simulink model "Saucer_4dof"  (R2015b)
settings: Solver=ode4  StartTime=0.0  StopTime=tsim  FixedStep=0.01  RelTol=1e-3
values from neighbouring files (symbols this model uses):
  eta_init = zeros(4,1)    [run_Saucer_4dof.m]
  nu_init = zeros(4,1)    [run_Saucer_4dof.m]
libraries: simulink x1
settings Model: Creator=mclab  LastModifiedBy=Rotem
settings DataIOCC: SaveFormat=Array
settings DebuggingCC: SolverPrmCheckMsg=warning
settings HardwareCC: ProdBitPerPointer=32  ProdLargestAtomicFloat=None  ProdIntDivRoundTo=Undefined  ProdEndianess=Unspecified  ProdWordSize=32  ProdHWDeviceType=32-bit Generic
settings RTWCC: SystemTargetFile=NIVeriStand_VxWorks.tlc  TemplateMakefile=NIVeriStand_VxWorks.tmf  Description=NI VeriStand VxWorks Real-Time Target for Release 2007b or later
settings STFCustomTargetCC: ConcurrentExecutionCompliant=off  MatFileLogging=on  MATLABClassNameForMDSCustomization=Simulink.SoftwareTarget.TargetSpecificTriggerConfigurationBase  CPPClassGenCompliant=off  SystemTargetFile=NIVeriStand_VxWorks.tlc
settings ConfigComp: CovModelRefEnable=Off  CovSFcnEnable=off

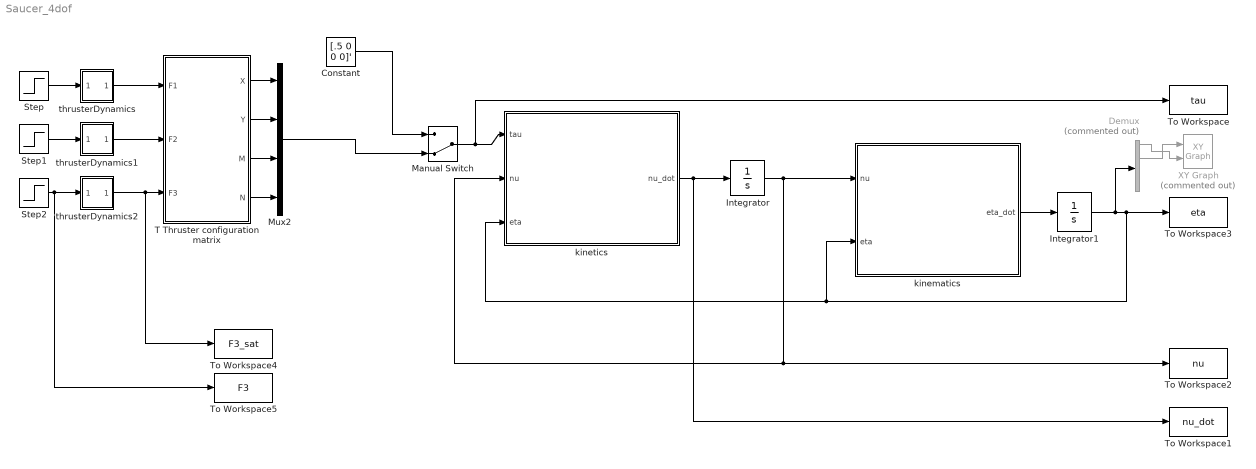
== system Saucer_4dof ==
  Constant : Constant  Value=[.5 0 0 0]'
  Demux : Demux  Commented=on
  Integrator : Integrator  InitialCondition=nu_init
  Integrator1 : Integrator  InitialCondition=eta_init
  Manual Switch : ManualSwitch  CurrentSetting=0
  Mux2 : Mux
  Step : Step  After=0  SampleTime=0  VectorParams1D=off
  Step1 : Step  After=.1  SampleTime=0  VectorParams1D=off
  Step2 : Step  After=-.1  SampleTime=0  VectorParams1D=off
  T Thruster configuration matrix : MATLAB Function  TreatAsAtomicUnit=on
  To Workspace : ToWorkspace  VariableName=tau  SaveFormat=Timeseries  SampleTime=-1
  To Workspace1 : ToWorkspace  VariableName=nu_dot  SaveFormat=Timeseries  SampleTime=-1
  To Workspace2 : ToWorkspace  VariableName=nu  SaveFormat=Timeseries  SampleTime=-1
  To Workspace3 : ToWorkspace  VariableName=eta  SaveFormat=Timeseries  SampleTime=-1
  To Workspace4 : ToWorkspace  VariableName=F3_sat  SaveFormat=Timeseries  SampleTime=-1
  To Workspace5 : ToWorkspace  VariableName=F3  SaveFormat=Timeseries  SampleTime=-1
  XY Graph : simulink/Sinks/XY Graph  Commented=on  xmin=-10  xmax=10  ymin=-10  ymax=10  st=-1
  kinematics : MATLAB Function  TreatAsAtomicUnit=on
  kinetics : MATLAB Function  TreatAsAtomicUnit=on
  thrusterDynamics : Subsystem
  thrusterDynamics1 : Subsystem
  thrusterDynamics2 : Subsystem
  wires:
  kinematics/1(eta_dot) -> Integrator1/1
  T Thruster configuration matrix/1(X) -> Mux2/1
  T Thruster configuration matrix/2(Y) -> Mux2/2
  Integrator/1 -> To Workspace2/1, kinetics/2(nu), kinematics/1(nu)
  T Thruster configuration matrix/4(N) -> Mux2/4
  T Thruster configuration matrix/3(M) -> Mux2/3
  thrusterDynamics/1(Out) -> T Thruster configuration matrix/1(F1)
  Integrator1/1 -> Demux/1, To Workspace3/1, kinetics/3(eta), kinematics/2(eta)
  thrusterDynamics1/1(Out) -> T Thruster configuration matrix/2(F2)
  Step1/1 -> thrusterDynamics1/1(In)
  Step2/1 -> thrusterDynamics2/1(In), To Workspace5/1
  thrusterDynamics2/1(Out) -> To Workspace4/1, T Thruster configuration matrix/3(F3)
  kinetics/1(nu_dot) -> To Workspace1/1, Integrator/1
  Step/1 -> thrusterDynamics/1(In)
  Manual Switch/1 -> To Workspace/1, kinetics/1(tau)
  Constant/1 -> Manual Switch/1
  Mux2/1 -> Manual Switch/2
  Demux/2 -> XY Graph/1
  Demux/1 -> XY Graph/2

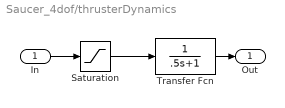
== system Saucer_4dof/thrusterDynamics ==
  In : Inport
  Saturation : Saturate  UpperLimit=4  LowerLimit=-4
  Transfer Fcn : TransferFcn  Denominator=[.5 1]
  Out : Outport
  wires:
  In/1 -> Saturation/1
  Transfer Fcn/1 -> Out/1
  Saturation/1 -> Transfer Fcn/1

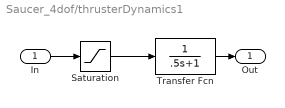
== system Saucer_4dof/thrusterDynamics1 ==
  In : Inport
  Saturation : Saturate  UpperLimit=4  LowerLimit=-4
  Transfer Fcn : TransferFcn  Denominator=[.5 1]
  Out : Outport
  wires:
  In/1 -> Saturation/1
  Transfer Fcn/1 -> Out/1
  Saturation/1 -> Transfer Fcn/1

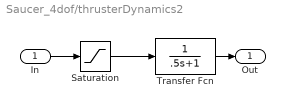
== system Saucer_4dof/thrusterDynamics2 ==
  In : Inport
  Saturation : Saturate  UpperLimit=4  LowerLimit=-4
  Transfer Fcn : TransferFcn  Denominator=[.5 1]
  Out : Outport
  wires:
  In/1 -> Saturation/1
  Transfer Fcn/1 -> Out/1
  Saturation/1 -> Transfer Fcn/1

== matlab function Saucer_4dof/kinematics ==
  data: nu input; eta_dot output; eta input
function eta_dot = Saucer_eta_dot(nu,eta)

%Getting the elements of eta
theta = eta(3);
psi = eta(4);
phi = 0; %Neglecting roll

%Finding the transformation matrix from {b} to {n}
[J6,J11,J22] = eulerang(phi,theta,psi);
J = J6([1,2,5,6],[1,2,5,6]); %Extracting relevant elements

eta_dot = J*nu;

== matlab function Saucer_4dof/kinetics ==
  data: tau input; nu_dot output; nu input; eta input
function nu_dot = Saucer_nu_dot(tau,nu,eta)

%To get column vectors (er dette nødvendig??)
nu = [nu(1);nu(2);nu(3);nu(4)];
tau = [tau(1);tau(2);tau(3);tau(4)];
%% PARAMETERS

% Physical constants and pendulum parameters:
g = 9.81; %Acceleration of gravity, m/s^2
rho = 1000; %Density of water, kg/m^3

%Vessel data:
m = 6.34; %Mass of the CS Saucer in kg
r = 0.548/2; %Radius of te CS Saucer
h = 0.129; %Total height of the CS Saucer
V = m/rho; %Volume displacement = mass displacement/rho
I_y = (1/12)*m*(3*r^2+h^2); %Mass moment of inertia about y axis (solid cylinder)
I_x = I_y;
% I_z = (m*r^2)/2;
I_z = 0.116; %From Idland (2015)
I_g = diag([I_x I_y I_z]); %Inertia tensor
r_g = [0 0 0]'; %Location of CG wrt CO
% r_b = [0 0 0.455]; %Location of CB wrt CO. Assuming B in centre of subm. vol.
% W = m*g; %Weight of the Saucer
% B = W; %Bouyancy

% Added mass:
X_dotu = -3.50; %Added mass in surge due to surge motion, kg
X_dotv = 0;
X_dotq = -0; %Added mass in surge due to motion in pitch
X_dotr = 0;
Y_dotu = X_dotv;
Y_dotv = X_dotu;
Y_dotq = 0;
Y_dotr = X_dotr;
M_dotu = -0;
M_dotv = 0;
M_dotq = -3; %Added mass in pitch due to pitch motion
M_dotr = 0;
N_dotu = 0;
N_dotv = 0;
N_dotq = 0;
N_dotr = 0;

% Damping:
X_u = -1.96; %Linear damping in surge due to surge motion
Y_v = -1.96;
M_q = -3; %Linear damping in pitch due to pitch motion
N_r = .1*X_u;
X_uu = -7.095; %Nonlinear damping in surge due to surge motion
Y_vv = -7.095;
M_qq = -12; %Nonlinear damping in pitch due to pitch motion
N_rr = 0.1*X_uu;

% Restoring:
I = (pi/4)*r^4; %Area moment of inertia
KG = (.129/2); %KG for the Saucer in m. Assuming it is in the centre
KB  = 0.038/2; %KB assuming it is in the centre of submerged volume
BM = I/V; %BM_L = BM_T
BG = KG-KB; %BM
GM = BM-BG; %GM (GM_L = GM_T)

%% MATRICES
% NB: For now values are taken from Ch. 2.4 in the project or guessed

%Mass:
M_RB = [m*eye(3) -m*Smtrx(r_g);
        m*Smtrx(r_g) I_g];
M_A = -[X_dotu X_dotv X_dotq X_dotr;
        Y_dotu Y_dotv Y_dotq Y_dotr;
        M_dotu M_dotv M_dotq M_dotr;
        N_dotu N_dotv N_dotq N_dotr];
    
M = M_RB([1 2 5 6],[1 2 5 6]) + M_A; %4DOF mass     
M6 = zeros(6); %Creating a 6 by 6 mass matrix, 6DOF mass
M6([1 2 5 6],[1 2 5 6]) = M; %Inserting the relevant mass in the 6 by 6 matrix

%Restoring:
gn = [0 0 rho*g*V*GM*sin(eta(3)) 0]'; %4 DOF restoring, Fossen. p. 64

%Linear + nonlinear damping matrix, uncoupled motion:
D_L = -diag([X_u,Y_v,M_q,N_r]);
D_NL= -diag([X_uu*abs(nu(1)),Y_vv*abs(nu(2)),M_qq*abs(nu(3)),N_rr*abs(nu(4))]);
D = D_L + D_NL;

%Coriolis:
nu6=[nu(1) nu(2) 0 0 nu(3) nu(4)]';
Cor6 = m2c(M6,nu6); %Fossen p.180 
C = Cor6([1 2 5 6],[1 2 5 6]); %Relevant Corliolis, surge and pitch

%% CALCULATION
nu_dot = M\(tau-(C+D)*nu-gn);

== matlab function Saucer_4dof/T Thruster configuration matrix ==
  data: F1 input; X output; F2 input; F3 input; Y output; M output; N output
function [X, Y, M, N] = fcn(F1,F2,F3)
%Gives the forces and moments as output, input being the force from each
%motor.

rt = 0.135; %Radius from CG to motor axis in m
l_z = 0.1; %Moment arm in pitch (m)

u = [F1 F2 F3]'; %Control input (positive clockwise)

%Thrust configuration matrix, fixed azimuth angles (120 deg)
Tr=[0 sin(2*pi/3) sin(4*pi/3);1 cos(2*pi/3) cos(4*pi/3);rt rt rt];

tau = Tr*u; 

X = tau(1);
Y = tau(2);
N = tau(3);
M = X*l_z; %Moment in pitch
